simulink model "untitled1"  (R2020b)
settings: Solver=FixedStepAuto  StartTime=0.0  StopTime=30  FixedStep=0.001  RelTol=1e-3
values from neighbouring files (symbols this model uses):
  C_D = 0.2    [Point_Mass.m]    (also in Point_mass_fancy_results.m = 0.6; point_mass_MAIN.m = 0.02; point_mass_unit_test_func.m = C_D; point_mass_verification.m)
  g = theta_dd_0*theta_d_0*cos(theta_0)*I_xy - phi_d_0*(theta_d_0)^2*sin(theta_0)*I_xy - phi_dd_0*theta_d_0*sin(theta_0)*I_xz - theta_d_0^2 * cos(theta_0)*I_xz + phi_d_0 * I_zx * theta_d_0 * cos(theta_0) + I_zy*phi_d_0^2*theta_d_0*sin(2*theta_0) + I_zz*phi_d_0 * theta_d_0 * cos(2*theta_0) + phi_d_0 * theta_d_0 * I_yx * sin(theta_0) - phi_d_0^2 * I_yy * theta_d_0 * cos(2*theta_0) + phi_d_0^2 * theta_d_0  ...(+23 chars)    [Gyro.m]    (also in Point_Mass.m = 9.81; Point_mass_fancy_results.m = 9.81; Tdt.m = cos(phi)*sin(theta)*cos(psi) + sin(phi)*sin(psi); angular_tune.m = (I_yx*I_zy - I_yy*I_zx)*(I_zx*wy_0 - I_yx*wz_0) + (I_xy*I_zx)
  m = theta_d_0*cos(theta_0)*I_yy - theta_d_0*sin(theta_0)*I_yz + I_xx*cos(theta_0)*theta_d_0 + 2*phi_d_0*I_xy*cos(theta_0)*sin(theta_0) + 2*phi_d_0*I_xz*(cos(theta_0))^2 - theta_d_0 * I_zy * sin(theta_0) - theta_d_0*cos(theta_0)*I_zz    [Gyro.m]    (also in Point_Mass.m = 100; Point_mass_fancy_results.m = 600; point_mass_MAIN.m = 640; point_mass_unit_test_func.m = mass)
  noise_power = 0.000000001    (= 1e-09)    [Point_mass_fancy_results.m]    (also in point_mass_MAIN.m; point_mass_verification.m = 0)
  rho = 0.991    [Point_Mass.m]    (also in Point_mass_fancy_results.m = 1.225; point_mass_MAIN.m = 1.225; point_mass_unit_test_func.m = density; point_mass_verification.m = 1.225)
  S = 4.5    [Point_Mass.m]    (also in Point_mass_fancy_results.m = 1.8; point_mass_MAIN.m = 2; point_mass_unit_test_func.m = S; point_mass_verification.m = 2)
  T = 10.5    [Point_mass_fancy_results.m]    (also in point_mass_MAIN.m; point_mass_unit_test_func.m = T; point_mass_verification.m = 1.5; six.m)
  time_delay = 0.3    [Point_mass_fancy_results.m]    (also in point_mass_MAIN.m = 3e-05; point_mass_unit_test_func.m = time_delay; point_mass_verification.m = 0.1; six.m = 0.1)
libraries: simulink x1, pid_lib x1
settings Model: Creator=Jonathan van Zyl  LastModifiedBy=Jonathan van Zyl

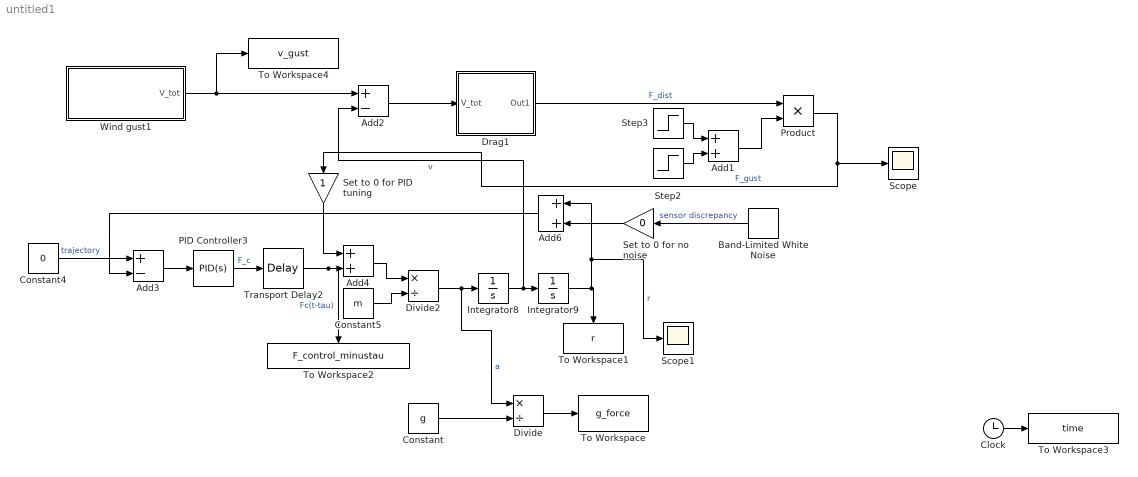
== system untitled1 ==
  Add1 : Sum
  Add2 : Sum  Inputs=+-
  Add3 : Sum  Inputs=+-
  Add4 : Sum
  Add6 : Sum
  Band-Limited White Noise : simulink/Sources/Band-Limited White Noise  Cov=[noise_power]  Ts=0.1  seed=[23341]
  Clock : Clock
  Constant : Constant  Value=g
  Constant4 : Constant  Value=0
  Constant5 : Constant  Value=m
  Divide : Product  Inputs=*/
  Divide2 : Product  Inputs=*/
  Drag1 : Subsystem
  Integrator8 : Integrator
  Integrator9 : Integrator
  PID Controller3 : pid_lib/PID Controller  Controller=PID  Form=Parallel  TimeDomain=Continuous-time  UseExternalTs=off  SampleTime=-1  IntegratorMethod=Forward Euler  FilterMethod=Forward Euler  ControllerParametersSource=internal  P=375  I=2.5080869601386  D=635.831408940251  UseFilter=on  N=114.28279760416  TunerSelectOption=Transfer Function Based (PID Tuner App)  InitialConditionSource=internal  InitialConditionForIntegrator=0  InitialConditionForFilter=0  DifferentiatorICPrevScaledInput=0  ExternalReset=none  TrackingMode=off  Kt=1  LimitOutput=off  SatLimitsSource=internal  UpperSaturationLimit=inf  LowerSaturationLimit=-inf  LinearizeAsGain=on  AntiWindupMode=none  Kb=1  POutMin=[]  POutMax=[]  IOutMin=[]  IOutMax=[]  DOutMin=[]  DOutMax=[]  NOutMin=[]  NOutMax=[]  SumOutMin=[]  SumOutMax=[]  SaturationOutMin=[]  SaturationOutMax=[]  PParamMin=[]  PParamMax=[]  IParamMin=[]  IParamMax=[]  DParamMin=[]  DParamMax=[]  NParamMin=[]  NParamMax=[]  KbParamMin=[]  KbParamMax=[]  KtParamMin=[]  KtParamMax=[]  KbOutMin=[]  KbOutMax=[]  KtOutMin=[]  KtOutMax=[]  IntegratorOutMin=[]  IntegratorOutMax=[]  FilterOutMin=[]  FilterOutMax=[]  SumI1OutMin=[]  SumI1OutMax=[]  SumI2OutMin=[]  SumI2OutMax=[]  SumI3OutMin=[]  SumI3OutMax=[]  SumI4OutMin=[]  SumI4OutMax=[]  SumDOutMin=[]  SumDOutMax=[]  DifferentiatorOutMin=[]  DifferentiatorOutMax=[]  FilterDiffOutCoefMin=[]  FilterDiffOutCoefMax=[]  ReciprocalOutMin=[]  ReciprocalOutMax=[]  SumDenOutMin=[]  SumDenOutMax=[]  SumNumOutMin=[]  SumNumOutMax=[]  DivideOutMin=[]  DivideOutMax=[]  UdiffTsProdOutMin=[]  UdiffTsProdOutMax=[]  NTsProdOutMin=[]  NTsProdOutMax=[]  UintegralTsProdOutMin=[]  UintegralTsProdOutMax=[]  UngainTsProdOutMin=[]  UngainTsProdOutMax=[]  IntegratorContinuousStateAttributes=''  IntegratorStateMustResolveToSignalObject=off  IntegratorRTWStateStorageClass=Auto  FilterContinuousStateAttributes=''  FilterStateMustResolveToSignalObject=off  FilterRTWStateStorageClass=Auto  ParallelPVariant=InternalParameters  IdealPVariant=Disabled  IVariant=InternalParameters  DVariant=InternalParameters  IntegratorVariant=Continuous  SatVariant=Disabled  AWVariant=Passthrough  PCopyVariant=Disabled  TRVariant=Disabled  FdbkBlocksVariant=Forward  IdealPFdbkVariant=Disabled  SatFdbkVariant=Disabled  DerivativeFilterVariant=ContFilter  NVariant=InternalParameters  NCopyVariant=Disabled  FilterICVariant=InternalICsFilter  IntegratorICVariant=InternalICs  ExternalResetVariant=Disabled  TRSumVariant=Passthrough  SumFdbkVariant=Disabled  SumVariant=Sum_PID  TsampFilterVariant=InternalTs  TsampNgainVariant=Passthrough  TsampIntegralVariant=Passthrough  ExternalSaturationOutDataTypeStr=Inherit: Same as second input
  Product : Product
  Scope : Scope
  Scope1 : Scope
  Set to 0 for PID tuning : Gain
  Set to 0 for no noise : Gain  Gain=0
  Step2 : Step  Time=0  SampleTime=0
  Step3 : Step  Time=10.5  After=-1  SampleTime=0
  To Workspace : ToWorkspace  VariableName=g_force  SaveFormat=Timeseries  SampleTime=-1
      settings: Save2DSignal=2-D array (concatenate along first dimension)
  To Workspace1 : ToWorkspace  VariableName=r  SaveFormat=Timeseries  SampleTime=-1
  To Workspace2 : ToWorkspace  VariableName=F_control_minustau  SaveFormat=Timeseries  SampleTime=-1
  To Workspace3 : ToWorkspace  VariableName=time  SaveFormat=Structure  SampleTime=-1
      settings: Save2DSignal=2-D array (concatenate along first dimension)
  To Workspace4 : ToWorkspace  VariableName=v_gust  SaveFormat=Timeseries  SampleTime=-1
  Transport Delay2 : TransportDelay  DelayTime=time_delay  TransDelayFeedthrough=on
  Wind gust1 : Subsystem
  wires:
  Constant4/1 -> Add3/1  "trajectory"
  Add3/1 -> PID Controller3/1
  PID Controller3/1 -> Transport Delay2/1  "F_c"
  Add4/1 -> Divide2/1
  Constant5/1 -> Divide2/2
  Divide2/1 -> Divide/1, Integrator8/1  "a"
  Integrator8/1 -> Add2/2, Integrator9/1  "v"
  Integrator9/1 -> Scope1/1, Add6/1, To Workspace1/1  "r"
  Drag1/1(Out1) -> Product/1  "F_dist"
  Transport Delay2/1 -> To Workspace2/1, Add4/2  "Fc(t-tau)"
  Band-Limited White Noise/1 -> Set to 0 for no noise/1  "sensor discrepancy"
  Add6/1 -> Add3/2
  Wind gust1/1(V_tot) -> To Workspace4/1, Add2/1
  Step3/1 -> Add1/1
  Step2/1 -> Add1/2
  Add1/1 -> Product/2
  Add2/1 -> Drag1/1(V_tot)
  Constant/1 -> Divide/2
  Divide/1 -> To Workspace/1
  Clock/1 -> To Workspace3/1
  Product/1 -> Scope/1, Set to 0 for PID tuning/1  "F_gust"
  Set to 0 for PID tuning/1 -> Add4/1
  Set to 0 for no noise/1 -> Add6/2

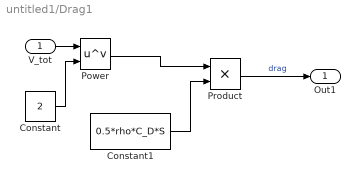
== system untitled1/Drag1 ==
  V_tot : Inport
  Constant : Constant  Value=2
  Constant1 : Constant  Value=0.5*rho*C_D*S
  Power : Math  Operator=pow  SaturateOnIntegerOverflow=on
  Product : Product
  Out1 : Outport
  wires:
  Constant1/1 -> Product/2
  Product/1 -> Out1/1  "drag"
  Constant/1 -> Power/2
  V_tot/1 -> Power/1
  Power/1 -> Product/1

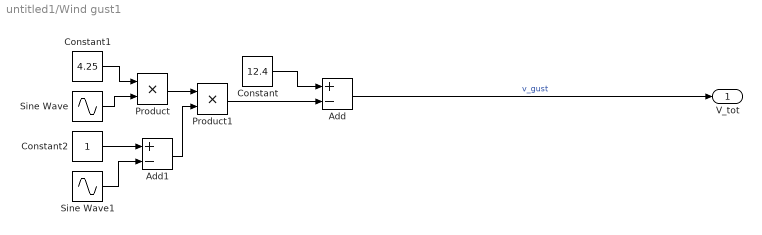
== system untitled1/Wind gust1 ==
  Add : Sum  Inputs=+-
  Add1 : Sum  Inputs=+-
  Constant : Constant  Value=12.4
  Constant1 : Constant  Value=4.25
  Constant2 : Constant
  Product : Product
  Product1 : Product
  Sine Wave : Sin  Frequency=3*pi/T  SampleTime=0
  Sine Wave1 : Sin  Frequency=2*pi/T  Phase=pi/2  SampleTime=0
  V_tot : Outport
  wires:
  Constant/1 -> Add/1
  Constant1/1 -> Product/1
  Sine Wave/1 -> Product/2
  Constant2/1 -> Add1/1
  Sine Wave1/1 -> Add1/2
  Product/1 -> Product1/1
  Add1/1 -> Product1/2
  Product1/1 -> Add/2
  Add/1 -> V_tot/1  "v_gust"
